simulink model "course_task_scheme_2019a"  (R2019a)
settings: Solver=ode15s  StartTime=0.0  StopTime=10  RelTol=1e-10  AbsTol=1e-10
values from neighbouring files (symbols this model uses):
  A_O = [-kappa*a_3, g_2, 0, 0;        -kappa^2*a_2, 0, g_3, 0;        -kappa^3*a_1, 0, 0, 1;        -kappa^4*a_0, 0, 0, 0]    [additional_calculations.m]
  B = 0.006    [course_task_script.m]
  b_O = [0; 0; overline_b; 0]    [additional_calculations.m]
  dist_2_amp = 0    [course_task_script.m]
  dist_2_bias = 0    [course_task_script.m]
  dist_2_freq = 0    [course_task_script.m]
  dist_2_phase = 0    [course_task_script.m]
  dist_amp = 0    [course_task_script.m]
  dist_bias = 0    [course_task_script.m]
  dist_freq = 0    [course_task_script.m]
  dist_noise_mean = 0    [course_task_script.m]
  dist_noise_variance = 1e-1    (= 0.1)    [course_task_script.m]
  dist_noised = 0    [course_task_script.m]
  dist_phase = 0    [course_task_script.m]
  eta_0 = zeros(3, 1)    [course_task_script.m]
  F = [zeros(n_F - 1, 1), eye(n_F - 1, n_F - 1); F_n]    [additional_calculations.m]
  G = [zeros(n_F - 1, 1); 1]    [additional_calculations.m]
  Gamma = S_n - F_n    [additional_calculations.m]
  hat_xi_0 = [0; 0; 0]    [course_task_script.m]
  i_0 = [0; 0]    [course_task_script.m]
  j = 0.55367e-4    (= 5.5367e-05)    [course_task_script.m]
  K = -poly_K(end:-1:2)    [additional_calculations.m]
  L = 20e-3    (= 0.02)    [course_task_script.m]
  L_O = g_2 * [kappa*a_3; kappa^2*a_2; kappa^3*a_1; kappa^4*a_0]    [additional_calculations.m]
  lambda_m = 0.06    [course_task_script.m]
  N = 1e+7    (= 10000000)    [course_task_script.m]
  n_p = 8    [course_task_script.m]
  noise_sample_time = 1e-3    (= 0.001)    [course_task_script.m]
  omega_0 = 0    [course_task_script.m]
  out_noise_mean = 0    [course_task_script.m]
  out_noise_variance = 1e-3    (= 0.001)    [course_task_script.m]
  out_noised = 0    [course_task_script.m]
  overline_b = 20    [course_task_script.m]
  R = 7.2    [course_task_script.m]
  sigma_0 = 0    [course_task_script.m]
  theta_0 = 0    [course_task_script.m]
  theta_ref = pi/3    (= 1.0471975512)    [course_task_script.m]
settings Model: Creator=hamme  LastModifiedBy=hamme
settings DebuggingCC: SFMachineParentedDataDiag=error

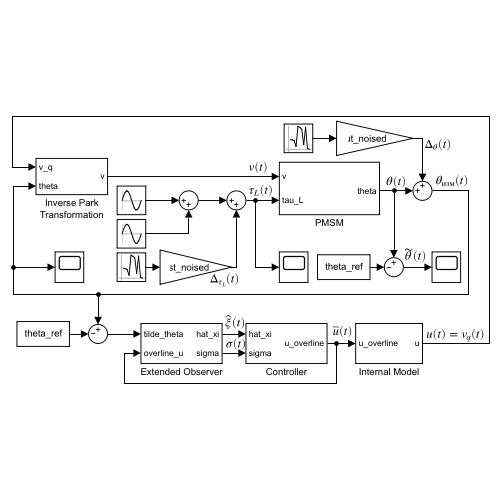
[thumbnail: Simulink's stored preview of the top-level diagram]
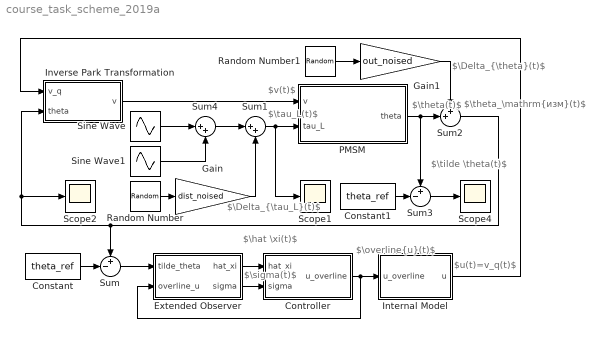
== system course_task_scheme_2019a ==
  note: $\tilde \theta(t)$
  note: $\hat \xi(t)$
  note: $\sigma(t)$
  note: $\overline{u}(t)$
  note: $u(t)=v_q(t)$
  note: $\tau_L(t)$
  note: $v(t)$
  note: $\theta(t)$
  note: $\theta_\mathrm{изм}(t)$
  note: $\Delta_{\tau_L}(t)$
  note: $\Delta_{\theta}(t)$
  Constant : Constant  Value=theta_ref
  Constant1 : Constant  Value=theta_ref
  Controller : Subsystem
  Extended Observer : Subsystem
  Gain : Gain  Gain=dist_noised
  Gain1 : Gain  Gain=out_noised
  Internal Model : Subsystem
  Inverse Park Transformation : Subsystem
  PMSM : Subsystem
  Random Number : RandomNumber  Mean=dist_noise_mean  Variance=dist_noise_variance  SampleTime=noise_sample_time
  Random Number1 : RandomNumber  Mean=out_noise_mean  Variance=out_noise_variance  SampleTime=noise_sample_time
  Scope1 : Scope
  Scope2 : Scope
  Scope4 : Scope
  Sine Wave : Sin  Amplitude=dist_amp  Bias=dist_bias  Frequency=dist_freq  Phase=dist_phase  SampleTime=0
  Sine Wave1 : Sin  Amplitude=dist_2_amp  Bias=dist_2_bias  Frequency=dist_2_freq  Phase=dist_2_phase  SampleTime=0
  Sum : Sum  Inputs=+-|
  Sum1 : Sum  Inputs=|++
  Sum2 : Sum  Inputs=++|
  Sum3 : Sum  Inputs=+-|
  Sum4 : Sum  Inputs=|++
  wires:
  PMSM/1(theta) -> Sum2/2, Sum3/1
  Constant/1 -> Sum/2
  Sum/1 -> Extended Observer/1(tilde_theta)
  Extended Observer/1(hat_xi) -> Controller/1(hat_xi)
  Extended Observer/2(sigma) -> Controller/2(sigma)
  Controller/1(u_overline) -> Extended Observer/2(overline_u), Internal Model/1(u_overline)
  Inverse Park Transformation/1(v) -> PMSM/1(v)
  Internal Model/1(u) -> Inverse Park Transformation/1(v_q)
  Random Number/1 -> Gain/1
  Sum1/1 -> Scope1/1, PMSM/2(tau_L)
  Gain/1 -> Sum1/2
  Random Number1/1 -> Gain1/1
  Gain1/1 -> Sum2/1
  Sum2/1 -> Inverse Park Transformation/2(theta), Scope2/1, Sum/1
  Constant1/1 -> Sum3/2
  Sum3/1 -> Scope4/1
  Sine Wave/1 -> Sum4/1
  Sum4/1 -> Sum1/1
  Sine Wave1/1 -> Sum4/2

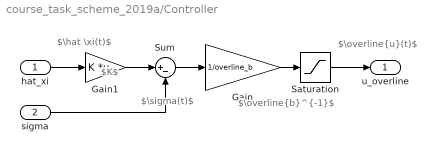
== system course_task_scheme_2019a/Controller ==
  note: $\hat \xi(t)$
  note: $\sigma(t)$
  note: $K$
  note: $\overline{b}^{-1}$
  note: $\overline{u}(t)$
  hat_xi : Inport
  sigma : Inport  Port=2
  Gain : Gain  Gain=1/overline_b
  Gain1 : Gain  Gain=K  Multiplication=Matrix(K*u)
  Saturation : Saturate  UpperLimit=N  LowerLimit=-N
  Sum : Sum  Inputs=|+-
  u_overline : Outport
  wires:
  Gain1/1 -> Sum/1
  hat_xi/1 -> Gain1/1
  sigma/1 -> Sum/2
  Sum/1 -> Gain/1
  Gain/1 -> Saturation/1
  Saturation/1 -> u_overline/1

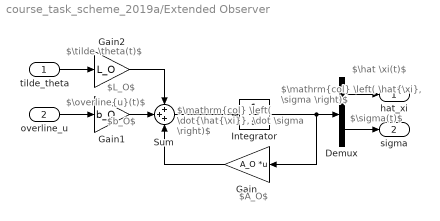
== system course_task_scheme_2019a/Extended Observer ==
  note: $A_O$
  note: $b_O$
  note: $L_O$
  note: $\mathrm{col} \left( \hat{\xi}, \sigma \right)$
  note: $\mathrm{col} \left( \dot{\hat{\xi}}, \dot \sigma \right)$
  note: $\hat \xi(t)$
  note: $\sigma(t)$
  note: $\tilde \theta(t)$
  note: $\overline{u}(t)$
  tilde_theta : Inport
  overline_u : Inport  Port=2
  Demux : Demux  Outputs=[3; 1]
  Gain : Gain  Gain=A_O  Multiplication=Matrix(K*u)
  Gain1 : Gain  Gain=b_O
  Gain2 : Gain  Gain=L_O
  Integrator : Integrator  InitialCondition=[hat_xi_0; sigma_0]
  Sum : Sum  Inputs=+++
  hat_xi : Outport
  sigma : Outport  Port=2
  wires:
  Integrator/1 -> Gain/1, Demux/1
  Gain/1 -> Sum/3
  Sum/1 -> Integrator/1
  overline_u/1 -> Gain1/1
  Gain1/1 -> Sum/2
  tilde_theta/1 -> Gain2/1
  Gain2/1 -> Sum/1
  Demux/1 -> hat_xi/1
  Demux/2 -> sigma/1

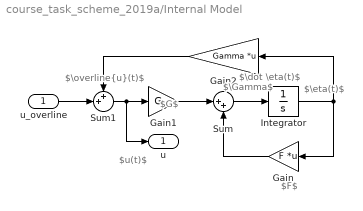
== system course_task_scheme_2019a/Internal Model ==
  note: $\Gamma$
  note: $F$
  note: $G$
  note: $\overline{u}(t)$
  note: $u(t)$
  note: $\eta(t)$
  note: $\dot \eta(t)$
  u_overline : Inport
  Gain : Gain  Gain=F  Multiplication=Matrix(K*u)
  Gain1 : Gain  Gain=G
  Gain2 : Gain  Gain=Gamma  Multiplication=Matrix(K*u)
  Integrator : Integrator  InitialCondition=eta_0
  Sum : Sum  Inputs=|++
  Sum1 : Sum  Inputs=++|
  u : Outport
  wires:
  Sum/1 -> Integrator/1
  Gain/1 -> Sum/2
  Integrator/1 -> Gain2/1, Gain/1
  u_overline/1 -> Sum1/2
  Gain1/1 -> Sum/1
  Sum1/1 -> u/1, Gain1/1
  Gain2/1 -> Sum1/1

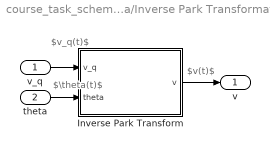
== system course_task_scheme_2019a/Inverse Park Transformation ==
  note: $v_q(t)$
  note: $\theta(t)$
  note: $v(t)$
  v_q : Inport
  theta : Inport  Port=2
  Inverse Park Transform : MATLAB Function  TreatAsAtomicUnit=on
  v : Outport
  wires:
  v_q/1 -> Inverse Park Transform/1(v_q)
  theta/1 -> Inverse Park Transform/2(theta)
  Inverse Park Transform/1(v) -> v/1

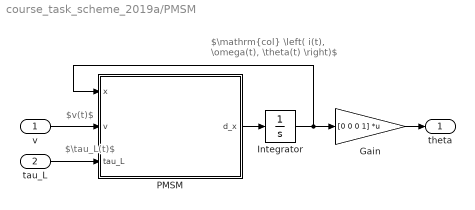
== system course_task_scheme_2019a/PMSM ==
  note: $v(t)$
  note: $\tau_L(t)$
  note: $\mathrm{col} \left( i(t), \omega(t), \theta(t) \right)$
  v : Inport
  tau_L : Inport  Port=2
  Gain : Gain  Gain=[0 0 0 1]  Multiplication=Matrix(K*u)
  Integrator : Integrator  InitialCondition=[ i_0; omega_0; theta_0 ]
  PMSM : MATLAB Function  TreatAsAtomicUnit=on
  theta : Outport
  wires:
  tau_L/1 -> PMSM/3(tau_L)
  v/1 -> PMSM/2(v)
  PMSM/1(d_x) -> Integrator/1
  Integrator/1 -> Gain/1, PMSM/1(x)
  Gain/1 -> theta/1

== matlab function course_task_scheme_2019a/PMSM/PMSM ==
  data: x input; v input; tau_L input; d_x output; R parameter; L parameter; lambda_m parameter; n_p parameter; j parameter; B parameter
function d_x = pmsm(x, v, tau_L, R, L, lambda_m, n_p, j, B)

i = x(1:2);
omega = x(3);
theta = x(4);

C=[cos(n_p*theta); sin(n_p*theta)]; 
J=[0,-1;1,0];
dC=n_p*J*C;

dot_i_ab=(1 / L) * (-R * i - omega * lambda_m * dC + v);  
dot_omega=(1 / j) * (-B * omega + lambda_m * i' * dC - tau_L);
dot_theta = omega;

d_x=[dot_i_ab;dot_omega;dot_theta];

== matlab function course_task_scheme_2019a/Inverse Park Transformation/Inverse Park Transform ==
  data: v_q input; v output; theta input; n_p parameter
function v = inv_park(v_q, theta, n_p)

xi_1 = n_p * theta;
v_dq = [0; v_q];

v = [ cos(xi_1), -sin(xi_1); sin(xi_1), cos(xi_1) ] * v_dq;
